simulink model "CHE572_Seminar_Simulink"  (Simulink 7.3)
settings: Solver=ode45  StartTime=0.0  StopTime=1.3  RelTol=1e-3
libraries: cstblocks x1
settings Model: Creator=Leily  LastModifiedBy=Leily

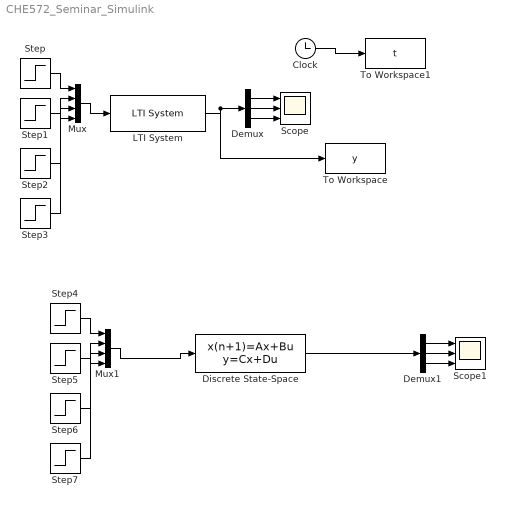
== system CHE572_Seminar_Simulink ==
  Clock : Clock
      settings: Decimation=10
  Demux : Demux  Outputs=3
  Demux1 : Demux  Outputs=3
  Discrete State-Space : DiscreteStateSpace  A=[0.3998 0;0 0.1599]  B=[0.6547 0 0.6547 0;-0.3749 45.8247 3.7493 4.5825]  C=[1 0; 0 1; 55 0]  D=zeros(3,4)  SampleTime=1/60
  LTI System : cstblocks/LTI System  SystemSampleTime=-1  sys=GpH  IC=[]
  Mux : Mux
  Mux1 : Mux
  Scope : Scope  NumInputPorts=3
      settings: YMin=-5~-5~-5  YMax=5~5~5
  Scope1 : Scope  NumInputPorts=3
      settings: YMin=-5~-5~-5  YMax=5~5~5
  Step : Step  Time=0  After=0  SampleTime=0
  Step1 : Step  Time=0  SampleTime=0
  Step{2..3,6..7} (4 alike) : Step  After=0  SampleTime=0
  Step4 : Step  Time=0  After=0  SampleTime=0
  Step5 : Step  Time=0  SampleTime=0
  To Workspace : ToWorkspace  VariableName=y  SampleTime=1/60  SaveFormat=Structure
  To Workspace1 : ToWorkspace  VariableName=t  SampleTime=1/60  SaveFormat=Structure
  wires:
  Mux/1 -> LTI System/1
  LTI System/1 -> Demux/1, To Workspace/1
  Demux/1 -> Scope/1
  Demux/2 -> Scope/2
  Demux/3 -> Scope/3
  Step/1 -> Mux/1
  Step1/1 -> Mux/2
  Step2/1 -> Mux/3
  Step3/1 -> Mux/4
  Mux1/1 -> Discrete State-Space/1
  Step4/1 -> Mux1/1
  Step5/1 -> Mux1/2
  Step6/1 -> Mux1/3
  Step7/1 -> Mux1/4
  Demux1/1 -> Scope1/1
  Demux1/2 -> Scope1/2
  Demux1/3 -> Scope1/3
  Discrete State-Space/1 -> Demux1/1
  Clock/1 -> To Workspace1/1
